simulink model "dc2dc"  (R2014a)
settings: Solver=ode45  StartTime=0.0  StopTime=Tmax  RelTol=1e-3
values from neighbouring files (symbols this model uses):
  Ac = [-1/p1, 0, 0 ... (first row only)    [array_init.m]
  Bc = [1/p1; p2/(p1*p3); (p4*p2)/(p1*p3*p5)]    [array_init.m]
  D = (Vref - Vs) / Vref    (= 0.6)    [array_init.m]
  T = 4e-6    (= 4e-06)    [array_init.m]
  Vs = 12    [array_init.m]
  Vs_noise = 0    [array_init.m]
undefined symbols (not defined in the file or in its folder): Ao, Bo
settings Model: Creator=Luan Nguyen  LastModifiedBy=Taylor
settings DataIOCC: SignalLoggingSaveFormat=ModelDataLogs
settings OptimizationCC: ExpressionDepthLimit=2147483647
settings DebuggingCC: UnderspecifiedInitializationDetection=Classic  MaxConsecutiveZCsMsg=none  MultiTaskDSMMsg=warning  MultiTaskCondExecSysMsg=none  StateNameClashWarn=warning
settings RTWCC: IncludeERTFirstTime=on

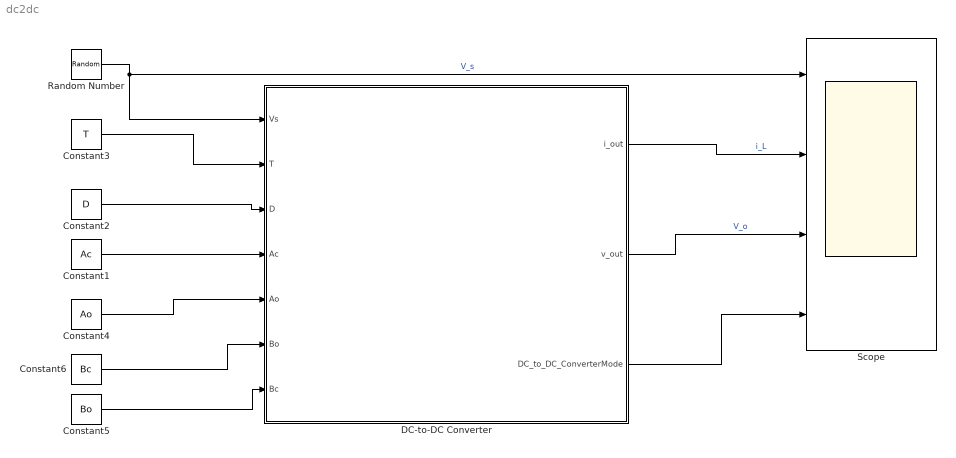
== system dc2dc ==
  Constant1 : Constant  Value=Ac
  Constant2 : Constant  Value=D
  Constant3 : Constant  Value=T
  Constant4 : Constant  Value=Ao
  Constant5 : Constant  Value=Bo
  Constant6 : Constant  Value=Bc
  DC-to-DC Converter : Stateflow chart  TreatAsAtomicUnit=on
  Random Number : RandomNumber  Mean=Vs  Variance=Vs_noise  SampleTime=T/10
  Scope : Scope  NumInputPorts=4
      settings: TimeRange=0.005  YMin=18~10.8827~17.91~1  YMax=18~10.8837~18.09~2
  wires:
  DC-to-DC Converter/1(i_out) -> Scope/2  "i_L"
  DC-to-DC Converter/2(v_out) -> Scope/3  "V_o"
  Constant2/1 -> DC-to-DC Converter/3(D)
  Constant3/1 -> DC-to-DC Converter/2(T)
  Random Number/1 -> Scope/1, DC-to-DC Converter/1(Vs)  "V_s"
  DC-to-DC Converter/3(DC_to_DC_ConverterMode) -> Scope/4
  Constant1/1 -> DC-to-DC Converter/4(Ac)
  Constant4/1 -> DC-to-DC Converter/5(Ao)
  Constant6/1 -> DC-to-DC Converter/6(Bo)
  Constant5/1 -> DC-to-DC Converter/7(Bc)

== stateflow chart dc2dc/DC-to-DC Converter ==
  settings: updateMethod=CONTINUOUS
  state Charging
    du:
    i_dot = Ac[0][0]*i+Ac[0][1]*v+Bc[0]*Vs;
    v_dot = Ac[1][0]*i+Ac[1][1]*v+Bc[1]*Vs;
    t_dot = 1;
    i_out = i;
    v_out = v;
  state Discharging
    du:
    i_dot = Ao[0][0]*i+Ao[0][1]*v+Bo[0]*Vs;
    v_dot = Ao[1][0]*i+Ao[1][1]*v+Bo[1]*Vs;
    t_dot = 1;
    i_out = i;
    v_out = v;
  Charging -> Discharging : [t>= D*T]
      | {t= 0;}
  Discharging -> Charging : [t>= (1-D)*T]
      | {t= 0;}
  (default) -> Discharging : {i = 0;
      | v = 0;}
  data: t local double; i_out output double; v_out output double; i local double; Vs input double =120; T input double; D input double; v local double; DC_to_DC_ConverterMode output Enum: DC_to_DC_ConverterModeType; Ac input double size=2,2; Ao input double size=2,2; Bo input double size=2,1; Bc input double size=2,1
  data t settings: updateMethod=SF_CONTINUOUS_TIME_DATA
  data i settings: updateMethod=SF_CONTINUOUS_TIME_DATA
  data v settings: updateMethod=SF_CONTINUOUS_TIME_DATA
